simulink model "Galton_Board_v2"  (R2021a)
settings: Solver=ode23t  StartTime=0.0  StopTime=10  MaxStep=1e-3  RelTol=1e-4  AbsTol=1e-4  EnableMultiTasking=on
PreLoadFcn:
  | init_Galton_Board;
values from neighbouring files (symbols this model uses):
  D_ball = 4    [init_Galton_Board.m]
  D_peg = 4    [init_Galton_Board.m]
  H_ground = 200    [init_Galton_Board.m]
  L_peg = 12    [init_Galton_Board.m]
  X = [29.5271269861 43.8447548606 71.2892627183 40.3733262692 -83.4271156395 -32.9172730858 85.8331450424 -78.3400144776 -42.6265382176 30.9682515097 40.2739041017 95.431354449 ... (500 elements, 1x500)]    [results.mat]
undefined symbols (not defined in the file or in its folder): Y, Z
libraries: sm_lib x965, nesl_utility x3
(part 3 of 3)

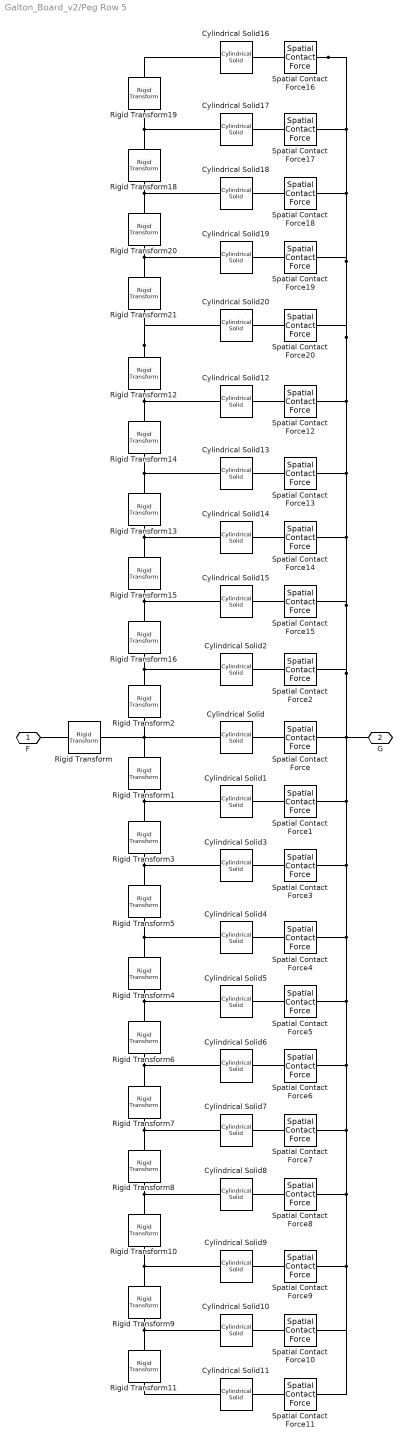
== system Galton_Board_v2/Peg Row 5 ==
  Cylindrical Solid{,1..20} (21 alike) : sm_lib/Body Elements/Cylindrical Solid  GraphicAmbientColor=[0.15 0.15 0.15 1.0]  BasedOnType=Density  CenterOfMass=[0 0 0]  CenterOfMassUnits=m  GraphicDiffuseColor=[0.5 0.5 0.5]  CylinderLength=D*4  CylinderLengthUnits=mm  CylinderRadius=D/2  CylinderRadiusUnits=mm  Density=1000  DensityUnits=kg/m^3  DoExposeReferenceFrame=on  GraphicEmissiveColor=[0.0 0.0 0.0 1.0]  ExportEntireGeometry=on  SerializedFrames=<Frames/>  MarkerShape=Sphere  MarkerSize=10  GraphicType=FromGeometry  InertiaType=CalculateFromGeometry  Mass=1  MassUnits=kg  MomentsOfInertia=[1 1 1]  MomentsOfInertiaUnits=kg*m^2  GraphicOpacity=1.0  ProductsOfInertia=[0 0 0]  ProductsOfInertiaUnits=kg*m^2  GraphicShininess=75  GraphicSpecularColor=[0.5 0.5 0.5 1.0]  GraphicVisPropType=SimpleVisualProperties
  Rigid Transform : sm_lib/Frames and Transforms/Rigid Transform  TranslationMethod=None  TranslationStandardOffset=0  TranslationLengthUnit=m  TranslationStandardAxis=+Z  TranslationCartesianOffset=[0 0 0]  TranslationROffset=0  TranslationROffsetUnits=m  TranslationZOffset=0  TranslationZOffsetUnits=m  TranslationThetaOffset=0  TranslationThetaOffsetUnits=deg  RotationMethod=StandardAxis  RotationAngleUnits=deg  RotationStandardAxis=+X  RotationAngle=90  RotationArbitraryAxis=[0 0 1]  FollAlignAxisA=+X  BaseAlignAxisA=+Y  FollAlignAxisB=+Y  BaseAlignAxisB=+Z  RotationSequenceAxes=FollowerAxes  RotationSequence=XYX  RotationSequenceAngles=[0 0 0]  RotationSequenceAnglesUnits=deg  RotationMatrix=[1 0 0; 0 1 0; 0 0 1]
  Rigid Transform{1..16,18..21} (20 alike) : sm_lib/Frames and Transforms/Rigid Transform  TranslationMethod=StandardAxis  TranslationStandardOffset=L  TranslationLengthUnit=mm  TranslationStandardAxis=+X  TranslationCartesianOffset=[0 0 0]  TranslationROffset=0  TranslationROffsetUnits=m  TranslationZOffset=0  TranslationZOffsetUnits=m  TranslationThetaOffset=0  TranslationThetaOffsetUnits=deg  RotationMethod=None  RotationAngleUnits=deg  RotationStandardAxis=+X  RotationAngle=90  RotationArbitraryAxis=[0 0 1]  FollAlignAxisA=+X  BaseAlignAxisA=+Y  FollAlignAxisB=+Y  BaseAlignAxisB=+Z  RotationSequenceAxes=FollowerAxes  RotationSequence=XYX  RotationSequenceAngles=[0 0 0]  RotationSequenceAnglesUnits=deg  RotationMatrix=[1 0 0; 0 1 0; 0 0 1]
  Spatial Contact Force{,1..20} (21 alike) : sm_lib/Forces and Torques/Spatial Contact Force  CoefficientOfDynamicFriction=0.3  CoefficientOfStaticFriction=0.5  SenseContactBaseRotation=off  SenseContactBaseTranslation=off  NormalDamping=b_scf  NormalDampingUnits=N/(m/s)  SenseContactFollowerRotation=off  SenseContactFollowerTranslation=off  SenseContactSignal=off  NormalStiffness=k_scf  NormalStiffnessUnits=N/m  FrictionalCriticalVelocity=1e-3  FrictionalCriticalVelocityUnits=m/s  ZeroCrossDetectContactStartAndEnd=off  FrictionType=SmoothStickSlip  SenseFrictionalForceMagnitude=off  SenseNormalForceMagnitude=off  NormalForceType=SmoothSpringDamper  SenseNormalVelocity=off  SenseSeparationDistance=off  SenseTangentialVelocity=off  SenseTangentialVelocityMagnitude=off  NormalTransitionRegionWidth=d_scf  NormalTransitionRegionWidthUnits=mm
  F : PMIOPort  Side=Left
  G : PMIOPort  Port=2  Side=Right
  connections:
  Spatial Contact Force19/LConn1 -- Cylindrical Solid19/LConn1
  Spatial Contact Force18/LConn1 -- Cylindrical Solid18/LConn1
  Spatial Contact Force20/LConn1 -- Cylindrical Solid20/LConn1
  Cylindrical Solid17/LConn1 -- Spatial Contact Force17/LConn1
  Spatial Contact Force16/LConn1 -- Cylindrical Solid16/LConn1
  Rigid Transform12/LConn1 -- Cylindrical Solid20/RConn1 -- Rigid Transform21/RConn1
  Rigid Transform20/RConn1 -- Rigid Transform21/LConn1 -- Cylindrical Solid19/RConn1
  Rigid Transform19/RConn1 -- Rigid Transform18/LConn1 -- Cylindrical Solid17/RConn1
  Rigid Transform19/LConn1 -- Cylindrical Solid16/RConn1
  Rigid Transform20/LConn1 -- Rigid Transform18/RConn1 -- Cylindrical Solid18/RConn1
  Spatial Contact Force12/LConn1 -- Cylindrical Solid12/LConn1
  Cylindrical Solid13/LConn1 -- Spatial Contact Force13/LConn1
  Spatial Contact Force14/LConn1 -- Cylindrical Solid14/LConn1
  Spatial Contact Force15/LConn1 -- Cylindrical Solid15/LConn1
  Rigid Transform15/RConn1 -- Rigid Transform16/LConn1 -- Cylindrical Solid15/RConn1
  Rigid Transform15/LConn1 -- Rigid Transform13/RConn1 -- Cylindrical Solid14/RConn1
  Rigid Transform14/RConn1 -- Rigid Transform13/LConn1 -- Cylindrical Solid13/RConn1
  Rigid Transform12/RConn1 -- Rigid Transform14/LConn1 -- Cylindrical Solid12/RConn1
  Spatial Contact Force8/LConn1 -- Cylindrical Solid8/LConn1
  Spatial Contact Force7/LConn1 -- Cylindrical Solid7/LConn1
  Spatial Contact Force10/LConn1 -- Cylindrical Solid10/LConn1
  Rigid Transform11/RConn1 -- Cylindrical Solid11/RConn1
  Cylindrical Solid9/LConn1 -- Spatial Contact Force9/LConn1
  Spatial Contact Force11/LConn1 -- Cylindrical Solid11/LConn1
  Rigid Transform11/LConn1 -- Rigid Transform9/RConn1 -- Cylindrical Solid10/RConn1
  Rigid Transform10/RConn1 -- Rigid Transform9/LConn1 -- Cylindrical Solid9/RConn1
  Rigid Transform8/RConn1 -- Rigid Transform10/LConn1 -- Cylindrical Solid8/RConn1
  Rigid Transform7/RConn1 -- Rigid Transform8/LConn1 -- Cylindrical Solid7/RConn1
  Spatial Contact Force6/LConn1 -- Cylindrical Solid6/LConn1
  Cylindrical Solid4/LConn1 -- Spatial Contact Force4/LConn1
  Rigid Transform7/LConn1 -- Rigid Transform6/RConn1 -- Cylindrical Solid6/RConn1
  Spatial Contact Force5/LConn1 -- Cylindrical Solid5/LConn1
  Rigid Transform4/RConn1 -- Rigid Transform6/LConn1 -- Cylindrical Solid5/RConn1
  Rigid Transform4/LConn1 -- Rigid Transform5/RConn1 -- Cylindrical Solid4/RConn1
  Rigid Transform5/LConn1 -- Rigid Transform3/RConn1 -- Cylindrical Solid3/RConn1
  Spatial Contact Force3/LConn1 -- Cylindrical Solid3/LConn1
  Rigid Transform16/RConn1 -- Cylindrical Solid2/RConn1 -- Rigid Transform2/LConn1
  Spatial Contact Force2/LConn1 -- Cylindrical Solid2/LConn1
  Spatial Contact Force1/LConn1 -- Cylindrical Solid1/LConn1
  Spatial Contact Force16/RConn1 -- Spatial Contact Force17/RConn1 -- Spatial Contact Force18/RConn1 -- Spatial Contact Force19/RConn1 -- Spatial Contact Force20/RConn1 -- Spatial Contact Force15/RConn1 -- Spatial Contact Force2/RConn1 -- Spatial Contact Force/RConn1 -- G/RConn1 -- Spatial Contact Force1/RConn1 -- Spatial Contact Force3/RConn1 -- Spatial Contact Force5/RConn1 -- Spatial Contact Force10/RConn1 -- Spatial Contact Force11/RConn1 -- Spatial Contact Force9/RConn1 -- Spatial Contact Force8/RConn1 -- Spatial Contact Force7/RConn1 -- Spatial Contact Force6/RConn1 -- Spatial Contact Force4/RConn1 -- Spatial Contact Force14/RConn1 -- Spatial Contact Force13/RConn1 -- Spatial Contact Force12/RConn1
  Rigid Transform3/LConn1 -- Rigid Transform1/RConn1 -- Cylindrical Solid1/RConn1
  Cylindrical Solid/LConn1 -- Spatial Contact Force/LConn1
  Rigid Transform/LConn1 -- F/RConn1
  Rigid Transform2/RConn1 -- Rigid Transform1/LConn1 -- Cylindrical Solid/RConn1 -- Rigid Transform/RConn1

== system Galton_Board_v2/Peg Row 6 ==
  Cylindrical Solid{,1..20} (21 alike) : sm_lib/Body Elements/Cylindrical Solid  GraphicAmbientColor=[0.15 0.15 0.15 1.0]  BasedOnType=Density  CenterOfMass=[0 0 0]  CenterOfMassUnits=m  GraphicDiffuseColor=[0.5 0.5 0.5]  CylinderLength=D*4  CylinderLengthUnits=mm  CylinderRadius=D/2  CylinderRadiusUnits=mm  Density=1000  DensityUnits=kg/m^3  DoExposeReferenceFrame=on  GraphicEmissiveColor=[0.0 0.0 0.0 1.0]  ExportEntireGeometry=on  SerializedFrames=<Frames/>  MarkerShape=Sphere  MarkerSize=10  GraphicType=FromGeometry  InertiaType=CalculateFromGeometry  Mass=1  MassUnits=kg  MomentsOfInertia=[1 1 1]  MomentsOfInertiaUnits=kg*m^2  GraphicOpacity=1.0  ProductsOfInertia=[0 0 0]  ProductsOfInertiaUnits=kg*m^2  GraphicShininess=75  GraphicSpecularColor=[0.5 0.5 0.5 1.0]  GraphicVisPropType=SimpleVisualProperties
  Rigid Transform : sm_lib/Frames and Transforms/Rigid Transform  TranslationMethod=None  TranslationStandardOffset=0  TranslationLengthUnit=m  TranslationStandardAxis=+Z  TranslationCartesianOffset=[0 0 0]  TranslationROffset=0  TranslationROffsetUnits=m  TranslationZOffset=0  TranslationZOffsetUnits=m  TranslationThetaOffset=0  TranslationThetaOffsetUnits=deg  RotationMethod=StandardAxis  RotationAngleUnits=deg  RotationStandardAxis=+X  RotationAngle=90  RotationArbitraryAxis=[0 0 1]  FollAlignAxisA=+X  BaseAlignAxisA=+Y  FollAlignAxisB=+Y  BaseAlignAxisB=+Z  RotationSequenceAxes=FollowerAxes  RotationSequence=XYX  RotationSequenceAngles=[0 0 0]  RotationSequenceAnglesUnits=deg  RotationMatrix=[1 0 0; 0 1 0; 0 0 1]
  Rigid Transform{1..16,18..21} (20 alike) : sm_lib/Frames and Transforms/Rigid Transform  TranslationMethod=StandardAxis  TranslationStandardOffset=L  TranslationLengthUnit=mm  TranslationStandardAxis=+X  TranslationCartesianOffset=[0 0 0]  TranslationROffset=0  TranslationROffsetUnits=m  TranslationZOffset=0  TranslationZOffsetUnits=m  TranslationThetaOffset=0  TranslationThetaOffsetUnits=deg  RotationMethod=None  RotationAngleUnits=deg  RotationStandardAxis=+X  RotationAngle=90  RotationArbitraryAxis=[0 0 1]  FollAlignAxisA=+X  BaseAlignAxisA=+Y  FollAlignAxisB=+Y  BaseAlignAxisB=+Z  RotationSequenceAxes=FollowerAxes  RotationSequence=XYX  RotationSequenceAngles=[0 0 0]  RotationSequenceAnglesUnits=deg  RotationMatrix=[1 0 0; 0 1 0; 0 0 1]
  Spatial Contact Force{,1..20} (21 alike) : sm_lib/Forces and Torques/Spatial Contact Force  CoefficientOfDynamicFriction=0.3  CoefficientOfStaticFriction=0.5  SenseContactBaseRotation=off  SenseContactBaseTranslation=off  NormalDamping=b_scf  NormalDampingUnits=N/(m/s)  SenseContactFollowerRotation=off  SenseContactFollowerTranslation=off  SenseContactSignal=off  NormalStiffness=k_scf  NormalStiffnessUnits=N/m  FrictionalCriticalVelocity=1e-3  FrictionalCriticalVelocityUnits=m/s  ZeroCrossDetectContactStartAndEnd=off  FrictionType=SmoothStickSlip  SenseFrictionalForceMagnitude=off  SenseNormalForceMagnitude=off  NormalForceType=SmoothSpringDamper  SenseNormalVelocity=off  SenseSeparationDistance=off  SenseTangentialVelocity=off  SenseTangentialVelocityMagnitude=off  NormalTransitionRegionWidth=d_scf  NormalTransitionRegionWidthUnits=mm
  F : PMIOPort  Side=Left
  G : PMIOPort  Port=2  Side=Right
  connections:
  Spatial Contact Force19/LConn1 -- Cylindrical Solid19/LConn1
  Spatial Contact Force18/LConn1 -- Cylindrical Solid18/LConn1
  Spatial Contact Force20/LConn1 -- Cylindrical Solid20/LConn1
  Cylindrical Solid17/LConn1 -- Spatial Contact Force17/LConn1
  Spatial Contact Force16/LConn1 -- Cylindrical Solid16/LConn1
  Rigid Transform12/LConn1 -- Cylindrical Solid20/RConn1 -- Rigid Transform21/RConn1
  Rigid Transform20/RConn1 -- Rigid Transform21/LConn1 -- Cylindrical Solid19/RConn1
  Rigid Transform19/RConn1 -- Rigid Transform18/LConn1 -- Cylindrical Solid17/RConn1
  Rigid Transform19/LConn1 -- Cylindrical Solid16/RConn1
  Rigid Transform20/LConn1 -- Rigid Transform18/RConn1 -- Cylindrical Solid18/RConn1
  Spatial Contact Force12/LConn1 -- Cylindrical Solid12/LConn1
  Cylindrical Solid13/LConn1 -- Spatial Contact Force13/LConn1
  Spatial Contact Force14/LConn1 -- Cylindrical Solid14/LConn1
  Spatial Contact Force15/LConn1 -- Cylindrical Solid15/LConn1
  Rigid Transform15/RConn1 -- Rigid Transform16/LConn1 -- Cylindrical Solid15/RConn1
  Rigid Transform15/LConn1 -- Rigid Transform13/RConn1 -- Cylindrical Solid14/RConn1
  Rigid Transform14/RConn1 -- Rigid Transform13/LConn1 -- Cylindrical Solid13/RConn1
  Rigid Transform12/RConn1 -- Rigid Transform14/LConn1 -- Cylindrical Solid12/RConn1
  Spatial Contact Force8/LConn1 -- Cylindrical Solid8/LConn1
  Spatial Contact Force7/LConn1 -- Cylindrical Solid7/LConn1
  Spatial Contact Force10/LConn1 -- Cylindrical Solid10/LConn1
  Rigid Transform11/RConn1 -- Cylindrical Solid11/RConn1
  Cylindrical Solid9/LConn1 -- Spatial Contact Force9/LConn1
  Spatial Contact Force11/LConn1 -- Cylindrical Solid11/LConn1
  Rigid Transform11/LConn1 -- Rigid Transform9/RConn1 -- Cylindrical Solid10/RConn1
  Rigid Transform10/RConn1 -- Rigid Transform9/LConn1 -- Cylindrical Solid9/RConn1
  Rigid Transform8/RConn1 -- Rigid Transform10/LConn1 -- Cylindrical Solid8/RConn1
  Rigid Transform7/RConn1 -- Rigid Transform8/LConn1 -- Cylindrical Solid7/RConn1
  Spatial Contact Force6/LConn1 -- Cylindrical Solid6/LConn1
  Cylindrical Solid4/LConn1 -- Spatial Contact Force4/LConn1
  Rigid Transform7/LConn1 -- Rigid Transform6/RConn1 -- Cylindrical Solid6/RConn1
  Spatial Contact Force5/LConn1 -- Cylindrical Solid5/LConn1
  Rigid Transform4/RConn1 -- Rigid Transform6/LConn1 -- Cylindrical Solid5/RConn1
  Rigid Transform4/LConn1 -- Rigid Transform5/RConn1 -- Cylindrical Solid4/RConn1
  Rigid Transform5/LConn1 -- Rigid Transform3/RConn1 -- Cylindrical Solid3/RConn1
  Spatial Contact Force3/LConn1 -- Cylindrical Solid3/LConn1
  Rigid Transform16/RConn1 -- Cylindrical Solid2/RConn1 -- Rigid Transform2/LConn1
  Spatial Contact Force2/LConn1 -- Cylindrical Solid2/LConn1
  Spatial Contact Force1/LConn1 -- Cylindrical Solid1/LConn1
  Spatial Contact Force16/RConn1 -- Spatial Contact Force17/RConn1 -- Spatial Contact Force18/RConn1 -- Spatial Contact Force19/RConn1 -- Spatial Contact Force20/RConn1 -- Spatial Contact Force15/RConn1 -- Spatial Contact Force2/RConn1 -- Spatial Contact Force/RConn1 -- G/RConn1 -- Spatial Contact Force1/RConn1 -- Spatial Contact Force3/RConn1 -- Spatial Contact Force5/RConn1 -- Spatial Contact Force10/RConn1 -- Spatial Contact Force11/RConn1 -- Spatial Contact Force9/RConn1 -- Spatial Contact Force8/RConn1 -- Spatial Contact Force7/RConn1 -- Spatial Contact Force6/RConn1 -- Spatial Contact Force4/RConn1 -- Spatial Contact Force14/RConn1 -- Spatial Contact Force13/RConn1 -- Spatial Contact Force12/RConn1
  Rigid Transform3/LConn1 -- Rigid Transform1/RConn1 -- Cylindrical Solid1/RConn1
  Cylindrical Solid/LConn1 -- Spatial Contact Force/LConn1
  Rigid Transform/LConn1 -- F/RConn1
  Rigid Transform2/RConn1 -- Rigid Transform1/LConn1 -- Cylindrical Solid/RConn1 -- Rigid Transform/RConn1

== system Galton_Board_v2/Peg Row 7 ==
  Cylindrical Solid{,1..20} (21 alike) : sm_lib/Body Elements/Cylindrical Solid  GraphicAmbientColor=[0.15 0.15 0.15 1.0]  BasedOnType=Density  CenterOfMass=[0 0 0]  CenterOfMassUnits=m  GraphicDiffuseColor=[0.5 0.5 0.5]  CylinderLength=D*4  CylinderLengthUnits=mm  CylinderRadius=D/2  CylinderRadiusUnits=mm  Density=1000  DensityUnits=kg/m^3  DoExposeReferenceFrame=on  GraphicEmissiveColor=[0.0 0.0 0.0 1.0]  ExportEntireGeometry=on  SerializedFrames=<Frames/>  MarkerShape=Sphere  MarkerSize=10  GraphicType=FromGeometry  InertiaType=CalculateFromGeometry  Mass=1  MassUnits=kg  MomentsOfInertia=[1 1 1]  MomentsOfInertiaUnits=kg*m^2  GraphicOpacity=1.0  ProductsOfInertia=[0 0 0]  ProductsOfInertiaUnits=kg*m^2  GraphicShininess=75  GraphicSpecularColor=[0.5 0.5 0.5 1.0]  GraphicVisPropType=SimpleVisualProperties
  Rigid Transform : sm_lib/Frames and Transforms/Rigid Transform  TranslationMethod=None  TranslationStandardOffset=0  TranslationLengthUnit=m  TranslationStandardAxis=+Z  TranslationCartesianOffset=[0 0 0]  TranslationROffset=0  TranslationROffsetUnits=m  TranslationZOffset=0  TranslationZOffsetUnits=m  TranslationThetaOffset=0  TranslationThetaOffsetUnits=deg  RotationMethod=StandardAxis  RotationAngleUnits=deg  RotationStandardAxis=+X  RotationAngle=90  RotationArbitraryAxis=[0 0 1]  FollAlignAxisA=+X  BaseAlignAxisA=+Y  FollAlignAxisB=+Y  BaseAlignAxisB=+Z  RotationSequenceAxes=FollowerAxes  RotationSequence=XYX  RotationSequenceAngles=[0 0 0]  RotationSequenceAnglesUnits=deg  RotationMatrix=[1 0 0; 0 1 0; 0 0 1]
  Rigid Transform{1..16,18..21} (20 alike) : sm_lib/Frames and Transforms/Rigid Transform  TranslationMethod=StandardAxis  TranslationStandardOffset=L  TranslationLengthUnit=mm  TranslationStandardAxis=+X  TranslationCartesianOffset=[0 0 0]  TranslationROffset=0  TranslationROffsetUnits=m  TranslationZOffset=0  TranslationZOffsetUnits=m  TranslationThetaOffset=0  TranslationThetaOffsetUnits=deg  RotationMethod=None  RotationAngleUnits=deg  RotationStandardAxis=+X  RotationAngle=90  RotationArbitraryAxis=[0 0 1]  FollAlignAxisA=+X  BaseAlignAxisA=+Y  FollAlignAxisB=+Y  BaseAlignAxisB=+Z  RotationSequenceAxes=FollowerAxes  RotationSequence=XYX  RotationSequenceAngles=[0 0 0]  RotationSequenceAnglesUnits=deg  RotationMatrix=[1 0 0; 0 1 0; 0 0 1]
  Spatial Contact Force{,1..20} (21 alike) : sm_lib/Forces and Torques/Spatial Contact Force  CoefficientOfDynamicFriction=0.3  CoefficientOfStaticFriction=0.5  SenseContactBaseRotation=off  SenseContactBaseTranslation=off  NormalDamping=b_scf  NormalDampingUnits=N/(m/s)  SenseContactFollowerRotation=off  SenseContactFollowerTranslation=off  SenseContactSignal=off  NormalStiffness=k_scf  NormalStiffnessUnits=N/m  FrictionalCriticalVelocity=1e-3  FrictionalCriticalVelocityUnits=m/s  ZeroCrossDetectContactStartAndEnd=off  FrictionType=SmoothStickSlip  SenseFrictionalForceMagnitude=off  SenseNormalForceMagnitude=off  NormalForceType=SmoothSpringDamper  SenseNormalVelocity=off  SenseSeparationDistance=off  SenseTangentialVelocity=off  SenseTangentialVelocityMagnitude=off  NormalTransitionRegionWidth=d_scf  NormalTransitionRegionWidthUnits=mm
  F : PMIOPort  Side=Left
  G : PMIOPort  Port=2  Side=Right
  connections:
  Rigid Transform/RConn1 -- Cylindrical Solid/RConn1 -- Rigid Transform1/LConn1 -- Rigid Transform2/RConn1
  Rigid Transform/LConn1 -- F/RConn1
  Cylindrical Solid/LConn1 -- Spatial Contact Force/LConn1
  Cylindrical Solid1/RConn1 -- Rigid Transform1/RConn1 -- Rigid Transform3/LConn1
  Spatial Contact Force12/RConn1 -- Spatial Contact Force13/RConn1 -- Spatial Contact Force14/RConn1 -- Spatial Contact Force4/RConn1 -- Spatial Contact Force6/RConn1 -- Spatial Contact Force7/RConn1 -- Spatial Contact Force8/RConn1 -- Spatial Contact Force9/RConn1 -- Spatial Contact Force11/RConn1 -- Spatial Contact Force10/RConn1 -- Spatial Contact Force5/RConn1 -- Spatial Contact Force3/RConn1 -- Spatial Contact Force1/RConn1 -- G/RConn1 -- Spatial Contact Force/RConn1 -- Spatial Contact Force2/RConn1 -- Spatial Contact Force15/RConn1 -- Spatial Contact Force20/RConn1 -- Spatial Contact Force19/RConn1 -- Spatial Contact Force18/RConn1 -- Spatial Contact Force17/RConn1 -- Spatial Contact Force16/RConn1
  Spatial Contact Force1/LConn1 -- Cylindrical Solid1/LConn1
  Spatial Contact Force2/LConn1 -- Cylindrical Solid2/LConn1
  Rigid Transform2/LConn1 -- Cylindrical Solid2/RConn1 -- Rigid Transform16/RConn1
  Spatial Contact Force3/LConn1 -- Cylindrical Solid3/LConn1
  Cylindrical Solid3/RConn1 -- Rigid Transform3/RConn1 -- Rigid Transform5/LConn1
  Cylindrical Solid4/RConn1 -- Rigid Transform5/RConn1 -- Rigid Transform4/LConn1
  Cylindrical Solid5/RConn1 -- Rigid Transform6/LConn1 -- Rigid Transform4/RConn1
  Spatial Contact Force5/LConn1 -- Cylindrical Solid5/LConn1
  Cylindrical Solid6/RConn1 -- Rigid Transform6/RConn1 -- Rigid Transform7/LConn1
  Cylindrical Solid4/LConn1 -- Spatial Contact Force4/LConn1
  Spatial Contact Force6/LConn1 -- Cylindrical Solid6/LConn1
  Cylindrical Solid7/RConn1 -- Rigid Transform8/LConn1 -- Rigid Transform7/RConn1
  Cylindrical Solid8/RConn1 -- Rigid Transform10/LConn1 -- Rigid Transform8/RConn1
  Cylindrical Solid9/RConn1 -- Rigid Transform9/LConn1 -- Rigid Transform10/RConn1
  Cylindrical Solid10/RConn1 -- Rigid Transform9/RConn1 -- Rigid Transform11/LConn1
  Spatial Contact Force11/LConn1 -- Cylindrical Solid11/LConn1
  Cylindrical Solid9/LConn1 -- Spatial Contact Force9/LConn1
  Rigid Transform11/RConn1 -- Cylindrical Solid11/RConn1
  Spatial Contact Force10/LConn1 -- Cylindrical Solid10/LConn1
  Spatial Contact Force7/LConn1 -- Cylindrical Solid7/LConn1
  Spatial Contact Force8/LConn1 -- Cylindrical Solid8/LConn1
  Cylindrical Solid12/RConn1 -- Rigid Transform14/LConn1 -- Rigid Transform12/RConn1
  Cylindrical Solid13/RConn1 -- Rigid Transform13/LConn1 -- Rigid Transform14/RConn1
  Cylindrical Solid14/RConn1 -- Rigid Transform13/RConn1 -- Rigid Transform15/LConn1
  Cylindrical Solid15/RConn1 -- Rigid Transform16/LConn1 -- Rigid Transform15/RConn1
  Spatial Contact Force15/LConn1 -- Cylindrical Solid15/LConn1
  Spatial Contact Force14/LConn1 -- Cylindrical Solid14/LConn1
  Cylindrical Solid13/LConn1 -- Spatial Contact Force13/LConn1
  Spatial Contact Force12/LConn1 -- Cylindrical Solid12/LConn1
  Cylindrical Solid18/RConn1 -- Rigid Transform18/RConn1 -- Rigid Transform20/LConn1
  Rigid Transform19/LConn1 -- Cylindrical Solid16/RConn1
  Cylindrical Solid17/RConn1 -- Rigid Transform18/LConn1 -- Rigid Transform19/RConn1
  Cylindrical Solid19/RConn1 -- Rigid Transform21/LConn1 -- Rigid Transform20/RConn1
  Rigid Transform21/RConn1 -- Cylindrical Solid20/RConn1 -- Rigid Transform12/LConn1
  Spatial Contact Force16/LConn1 -- Cylindrical Solid16/LConn1
  Cylindrical Solid17/LConn1 -- Spatial Contact Force17/LConn1
  Spatial Contact Force20/LConn1 -- Cylindrical Solid20/LConn1
  Spatial Contact Force18/LConn1 -- Cylindrical Solid18/LConn1
  Spatial Contact Force19/LConn1 -- Cylindrical Solid19/LConn1

== system Galton_Board_v2/Peg Row 8 ==
  Cylindrical Solid{,1..20} (21 alike) : sm_lib/Body Elements/Cylindrical Solid  GraphicAmbientColor=[0.15 0.15 0.15 1.0]  BasedOnType=Density  CenterOfMass=[0 0 0]  CenterOfMassUnits=m  GraphicDiffuseColor=[0.5 0.5 0.5]  CylinderLength=D*4  CylinderLengthUnits=mm  CylinderRadius=D/2  CylinderRadiusUnits=mm  Density=1000  DensityUnits=kg/m^3  DoExposeReferenceFrame=on  GraphicEmissiveColor=[0.0 0.0 0.0 1.0]  ExportEntireGeometry=on  SerializedFrames=<Frames/>  MarkerShape=Sphere  MarkerSize=10  GraphicType=FromGeometry  InertiaType=CalculateFromGeometry  Mass=1  MassUnits=kg  MomentsOfInertia=[1 1 1]  MomentsOfInertiaUnits=kg*m^2  GraphicOpacity=1.0  ProductsOfInertia=[0 0 0]  ProductsOfInertiaUnits=kg*m^2  GraphicShininess=75  GraphicSpecularColor=[0.5 0.5 0.5 1.0]  GraphicVisPropType=SimpleVisualProperties
  Rigid Transform : sm_lib/Frames and Transforms/Rigid Transform  TranslationMethod=None  TranslationStandardOffset=0  TranslationLengthUnit=m  TranslationStandardAxis=+Z  TranslationCartesianOffset=[0 0 0]  TranslationROffset=0  TranslationROffsetUnits=m  TranslationZOffset=0  TranslationZOffsetUnits=m  TranslationThetaOffset=0  TranslationThetaOffsetUnits=deg  RotationMethod=StandardAxis  RotationAngleUnits=deg  RotationStandardAxis=+X  RotationAngle=90  RotationArbitraryAxis=[0 0 1]  FollAlignAxisA=+X  BaseAlignAxisA=+Y  FollAlignAxisB=+Y  BaseAlignAxisB=+Z  RotationSequenceAxes=FollowerAxes  RotationSequence=XYX  RotationSequenceAngles=[0 0 0]  RotationSequenceAnglesUnits=deg  RotationMatrix=[1 0 0; 0 1 0; 0 0 1]
  Rigid Transform{1..16,18..21} (20 alike) : sm_lib/Frames and Transforms/Rigid Transform  TranslationMethod=StandardAxis  TranslationStandardOffset=L  TranslationLengthUnit=mm  TranslationStandardAxis=+X  TranslationCartesianOffset=[0 0 0]  TranslationROffset=0  TranslationROffsetUnits=m  TranslationZOffset=0  TranslationZOffsetUnits=m  TranslationThetaOffset=0  TranslationThetaOffsetUnits=deg  RotationMethod=None  RotationAngleUnits=deg  RotationStandardAxis=+X  RotationAngle=90  RotationArbitraryAxis=[0 0 1]  FollAlignAxisA=+X  BaseAlignAxisA=+Y  FollAlignAxisB=+Y  BaseAlignAxisB=+Z  RotationSequenceAxes=FollowerAxes  RotationSequence=XYX  RotationSequenceAngles=[0 0 0]  RotationSequenceAnglesUnits=deg  RotationMatrix=[1 0 0; 0 1 0; 0 0 1]
  Spatial Contact Force{,1..20} (21 alike) : sm_lib/Forces and Torques/Spatial Contact Force  CoefficientOfDynamicFriction=0.3  CoefficientOfStaticFriction=0.5  SenseContactBaseRotation=off  SenseContactBaseTranslation=off  NormalDamping=b_scf  NormalDampingUnits=N/(m/s)  SenseContactFollowerRotation=off  SenseContactFollowerTranslation=off  SenseContactSignal=off  NormalStiffness=k_scf  NormalStiffnessUnits=N/m  FrictionalCriticalVelocity=1e-3  FrictionalCriticalVelocityUnits=m/s  ZeroCrossDetectContactStartAndEnd=off  FrictionType=SmoothStickSlip  SenseFrictionalForceMagnitude=off  SenseNormalForceMagnitude=off  NormalForceType=SmoothSpringDamper  SenseNormalVelocity=off  SenseSeparationDistance=off  SenseTangentialVelocity=off  SenseTangentialVelocityMagnitude=off  NormalTransitionRegionWidth=d_scf  NormalTransitionRegionWidthUnits=mm
  F : PMIOPort  Side=Left
  G : PMIOPort  Port=2  Side=Right
  connections:
  Rigid Transform/RConn1 -- Cylindrical Solid/RConn1 -- Rigid Transform1/LConn1 -- Rigid Transform2/RConn1
  Rigid Transform/LConn1 -- F/RConn1
  Cylindrical Solid/LConn1 -- Spatial Contact Force/LConn1
  Cylindrical Solid1/RConn1 -- Rigid Transform1/RConn1 -- Rigid Transform3/LConn1
  Spatial Contact Force12/RConn1 -- Spatial Contact Force13/RConn1 -- Spatial Contact Force14/RConn1 -- Spatial Contact Force4/RConn1 -- Spatial Contact Force6/RConn1 -- Spatial Contact Force7/RConn1 -- Spatial Contact Force8/RConn1 -- Spatial Contact Force9/RConn1 -- Spatial Contact Force11/RConn1 -- Spatial Contact Force10/RConn1 -- Spatial Contact Force5/RConn1 -- Spatial Contact Force3/RConn1 -- Spatial Contact Force1/RConn1 -- G/RConn1 -- Spatial Contact Force/RConn1 -- Spatial Contact Force2/RConn1 -- Spatial Contact Force15/RConn1 -- Spatial Contact Force20/RConn1 -- Spatial Contact Force19/RConn1 -- Spatial Contact Force18/RConn1 -- Spatial Contact Force17/RConn1 -- Spatial Contact Force16/RConn1
  Spatial Contact Force1/LConn1 -- Cylindrical Solid1/LConn1
  Spatial Contact Force2/LConn1 -- Cylindrical Solid2/LConn1
  Rigid Transform2/LConn1 -- Cylindrical Solid2/RConn1 -- Rigid Transform16/RConn1
  Spatial Contact Force3/LConn1 -- Cylindrical Solid3/LConn1
  Cylindrical Solid3/RConn1 -- Rigid Transform3/RConn1 -- Rigid Transform5/LConn1
  Cylindrical Solid4/RConn1 -- Rigid Transform5/RConn1 -- Rigid Transform4/LConn1
  Cylindrical Solid5/RConn1 -- Rigid Transform6/LConn1 -- Rigid Transform4/RConn1
  Spatial Contact Force5/LConn1 -- Cylindrical Solid5/LConn1
  Cylindrical Solid6/RConn1 -- Rigid Transform6/RConn1 -- Rigid Transform7/LConn1
  Cylindrical Solid4/LConn1 -- Spatial Contact Force4/LConn1
  Spatial Contact Force6/LConn1 -- Cylindrical Solid6/LConn1
  Cylindrical Solid7/RConn1 -- Rigid Transform8/LConn1 -- Rigid Transform7/RConn1
  Cylindrical Solid8/RConn1 -- Rigid Transform10/LConn1 -- Rigid Transform8/RConn1
  Cylindrical Solid9/RConn1 -- Rigid Transform9/LConn1 -- Rigid Transform10/RConn1
  Cylindrical Solid10/RConn1 -- Rigid Transform9/RConn1 -- Rigid Transform11/LConn1
  Spatial Contact Force11/LConn1 -- Cylindrical Solid11/LConn1
  Cylindrical Solid9/LConn1 -- Spatial Contact Force9/LConn1
  Rigid Transform11/RConn1 -- Cylindrical Solid11/RConn1
  Spatial Contact Force10/LConn1 -- Cylindrical Solid10/LConn1
  Spatial Contact Force7/LConn1 -- Cylindrical Solid7/LConn1
  Spatial Contact Force8/LConn1 -- Cylindrical Solid8/LConn1
  Cylindrical Solid12/RConn1 -- Rigid Transform14/LConn1 -- Rigid Transform12/RConn1
  Cylindrical Solid13/RConn1 -- Rigid Transform13/LConn1 -- Rigid Transform14/RConn1
  Cylindrical Solid14/RConn1 -- Rigid Transform13/RConn1 -- Rigid Transform15/LConn1
  Cylindrical Solid15/RConn1 -- Rigid Transform16/LConn1 -- Rigid Transform15/RConn1
  Spatial Contact Force15/LConn1 -- Cylindrical Solid15/LConn1
  Spatial Contact Force14/LConn1 -- Cylindrical Solid14/LConn1
  Cylindrical Solid13/LConn1 -- Spatial Contact Force13/LConn1
  Spatial Contact Force12/LConn1 -- Cylindrical Solid12/LConn1
  Cylindrical Solid18/RConn1 -- Rigid Transform18/RConn1 -- Rigid Transform20/LConn1
  Rigid Transform19/LConn1 -- Cylindrical Solid16/RConn1
  Cylindrical Solid17/RConn1 -- Rigid Transform18/LConn1 -- Rigid Transform19/RConn1
  Cylindrical Solid19/RConn1 -- Rigid Transform21/LConn1 -- Rigid Transform20/RConn1
  Rigid Transform21/RConn1 -- Cylindrical Solid20/RConn1 -- Rigid Transform12/LConn1
  Spatial Contact Force16/LConn1 -- Cylindrical Solid16/LConn1
  Cylindrical Solid17/LConn1 -- Spatial Contact Force17/LConn1
  Spatial Contact Force20/LConn1 -- Cylindrical Solid20/LConn1
  Spatial Contact Force18/LConn1 -- Cylindrical Solid18/LConn1
  Spatial Contact Force19/LConn1 -- Cylindrical Solid19/LConn1

== system Galton_Board_v2/Peg Row 9 ==
  Cylindrical Solid{,1..20} (21 alike) : sm_lib/Body Elements/Cylindrical Solid  GraphicAmbientColor=[0.15 0.15 0.15 1.0]  BasedOnType=Density  CenterOfMass=[0 0 0]  CenterOfMassUnits=m  GraphicDiffuseColor=[0.5 0.5 0.5]  CylinderLength=D*4  CylinderLengthUnits=mm  CylinderRadius=D/2  CylinderRadiusUnits=mm  Density=1000  DensityUnits=kg/m^3  DoExposeReferenceFrame=on  GraphicEmissiveColor=[0.0 0.0 0.0 1.0]  ExportEntireGeometry=on  SerializedFrames=<Frames/>  MarkerShape=Sphere  MarkerSize=10  GraphicType=FromGeometry  InertiaType=CalculateFromGeometry  Mass=1  MassUnits=kg  MomentsOfInertia=[1 1 1]  MomentsOfInertiaUnits=kg*m^2  GraphicOpacity=1.0  ProductsOfInertia=[0 0 0]  ProductsOfInertiaUnits=kg*m^2  GraphicShininess=75  GraphicSpecularColor=[0.5 0.5 0.5 1.0]  GraphicVisPropType=SimpleVisualProperties
  Rigid Transform : sm_lib/Frames and Transforms/Rigid Transform  TranslationMethod=None  TranslationStandardOffset=0  TranslationLengthUnit=m  TranslationStandardAxis=+Z  TranslationCartesianOffset=[0 0 0]  TranslationROffset=0  TranslationROffsetUnits=m  TranslationZOffset=0  TranslationZOffsetUnits=m  TranslationThetaOffset=0  TranslationThetaOffsetUnits=deg  RotationMethod=StandardAxis  RotationAngleUnits=deg  RotationStandardAxis=+X  RotationAngle=90  RotationArbitraryAxis=[0 0 1]  FollAlignAxisA=+X  BaseAlignAxisA=+Y  FollAlignAxisB=+Y  BaseAlignAxisB=+Z  RotationSequenceAxes=FollowerAxes  RotationSequence=XYX  RotationSequenceAngles=[0 0 0]  RotationSequenceAnglesUnits=deg  RotationMatrix=[1 0 0; 0 1 0; 0 0 1]
  Rigid Transform{1..16,18..21} (20 alike) : sm_lib/Frames and Transforms/Rigid Transform  TranslationMethod=StandardAxis  TranslationStandardOffset=L  TranslationLengthUnit=mm  TranslationStandardAxis=+X  TranslationCartesianOffset=[0 0 0]  TranslationROffset=0  TranslationROffsetUnits=m  TranslationZOffset=0  TranslationZOffsetUnits=m  TranslationThetaOffset=0  TranslationThetaOffsetUnits=deg  RotationMethod=None  RotationAngleUnits=deg  RotationStandardAxis=+X  RotationAngle=90  RotationArbitraryAxis=[0 0 1]  FollAlignAxisA=+X  BaseAlignAxisA=+Y  FollAlignAxisB=+Y  BaseAlignAxisB=+Z  RotationSequenceAxes=FollowerAxes  RotationSequence=XYX  RotationSequenceAngles=[0 0 0]  RotationSequenceAnglesUnits=deg  RotationMatrix=[1 0 0; 0 1 0; 0 0 1]
  Spatial Contact Force{,1..20} (21 alike) : sm_lib/Forces and Torques/Spatial Contact Force  CoefficientOfDynamicFriction=0.3  CoefficientOfStaticFriction=0.5  SenseContactBaseRotation=off  SenseContactBaseTranslation=off  NormalDamping=b_scf  NormalDampingUnits=N/(m/s)  SenseContactFollowerRotation=off  SenseContactFollowerTranslation=off  SenseContactSignal=off  NormalStiffness=k_scf  NormalStiffnessUnits=N/m  FrictionalCriticalVelocity=1e-3  FrictionalCriticalVelocityUnits=m/s  ZeroCrossDetectContactStartAndEnd=off  FrictionType=SmoothStickSlip  SenseFrictionalForceMagnitude=off  SenseNormalForceMagnitude=off  NormalForceType=SmoothSpringDamper  SenseNormalVelocity=off  SenseSeparationDistance=off  SenseTangentialVelocity=off  SenseTangentialVelocityMagnitude=off  NormalTransitionRegionWidth=d_scf  NormalTransitionRegionWidthUnits=mm
  F : PMIOPort  Side=Left
  G : PMIOPort  Port=2  Side=Right
  connections:
  Spatial Contact Force19/LConn1 -- Cylindrical Solid19/LConn1
  Spatial Contact Force18/LConn1 -- Cylindrical Solid18/LConn1
  Spatial Contact Force20/LConn1 -- Cylindrical Solid20/LConn1
  Cylindrical Solid17/LConn1 -- Spatial Contact Force17/LConn1
  Spatial Contact Force16/LConn1 -- Cylindrical Solid16/LConn1
  Rigid Transform12/LConn1 -- Cylindrical Solid20/RConn1 -- Rigid Transform21/RConn1
  Rigid Transform20/RConn1 -- Rigid Transform21/LConn1 -- Cylindrical Solid19/RConn1
  Rigid Transform19/RConn1 -- Rigid Transform18/LConn1 -- Cylindrical Solid17/RConn1
  Rigid Transform19/LConn1 -- Cylindrical Solid16/RConn1
  Rigid Transform20/LConn1 -- Rigid Transform18/RConn1 -- Cylindrical Solid18/RConn1
  Spatial Contact Force12/LConn1 -- Cylindrical Solid12/LConn1
  Cylindrical Solid13/LConn1 -- Spatial Contact Force13/LConn1
  Spatial Contact Force14/LConn1 -- Cylindrical Solid14/LConn1
  Spatial Contact Force15/LConn1 -- Cylindrical Solid15/LConn1
  Rigid Transform15/RConn1 -- Rigid Transform16/LConn1 -- Cylindrical Solid15/RConn1
  Rigid Transform15/LConn1 -- Rigid Transform13/RConn1 -- Cylindrical Solid14/RConn1
  Rigid Transform14/RConn1 -- Rigid Transform13/LConn1 -- Cylindrical Solid13/RConn1
  Rigid Transform12/RConn1 -- Rigid Transform14/LConn1 -- Cylindrical Solid12/RConn1
  Spatial Contact Force8/LConn1 -- Cylindrical Solid8/LConn1
  Spatial Contact Force7/LConn1 -- Cylindrical Solid7/LConn1
  Spatial Contact Force10/LConn1 -- Cylindrical Solid10/LConn1
  Rigid Transform11/RConn1 -- Cylindrical Solid11/RConn1
  Cylindrical Solid9/LConn1 -- Spatial Contact Force9/LConn1
  Spatial Contact Force11/LConn1 -- Cylindrical Solid11/LConn1
  Rigid Transform11/LConn1 -- Rigid Transform9/RConn1 -- Cylindrical Solid10/RConn1
  Rigid Transform10/RConn1 -- Rigid Transform9/LConn1 -- Cylindrical Solid9/RConn1
  Rigid Transform8/RConn1 -- Rigid Transform10/LConn1 -- Cylindrical Solid8/RConn1
  Rigid Transform7/RConn1 -- Rigid Transform8/LConn1 -- Cylindrical Solid7/RConn1
  Spatial Contact Force6/LConn1 -- Cylindrical Solid6/LConn1
  Cylindrical Solid4/LConn1 -- Spatial Contact Force4/LConn1
  Rigid Transform7/LConn1 -- Rigid Transform6/RConn1 -- Cylindrical Solid6/RConn1
  Spatial Contact Force5/LConn1 -- Cylindrical Solid5/LConn1
  Rigid Transform4/RConn1 -- Rigid Transform6/LConn1 -- Cylindrical Solid5/RConn1
  Rigid Transform4/LConn1 -- Rigid Transform5/RConn1 -- Cylindrical Solid4/RConn1
  Rigid Transform5/LConn1 -- Rigid Transform3/RConn1 -- Cylindrical Solid3/RConn1
  Spatial Contact Force3/LConn1 -- Cylindrical Solid3/LConn1
  Rigid Transform16/RConn1 -- Cylindrical Solid2/RConn1 -- Rigid Transform2/LConn1
  Spatial Contact Force2/LConn1 -- Cylindrical Solid2/LConn1
  Spatial Contact Force1/LConn1 -- Cylindrical Solid1/LConn1
  Spatial Contact Force16/RConn1 -- Spatial Contact Force17/RConn1 -- Spatial Contact Force18/RConn1 -- Spatial Contact Force19/RConn1 -- Spatial Contact Force20/RConn1 -- Spatial Contact Force15/RConn1 -- Spatial Contact Force2/RConn1 -- Spatial Contact Force/RConn1 -- G/RConn1 -- Spatial Contact Force1/RConn1 -- Spatial Contact Force3/RConn1 -- Spatial Contact Force5/RConn1 -- Spatial Contact Force10/RConn1 -- Spatial Contact Force11/RConn1 -- Spatial Contact Force9/RConn1 -- Spatial Contact Force8/RConn1 -- Spatial Contact Force7/RConn1 -- Spatial Contact Force6/RConn1 -- Spatial Contact Force4/RConn1 -- Spatial Contact Force14/RConn1 -- Spatial Contact Force13/RConn1 -- Spatial Contact Force12/RConn1
  Rigid Transform3/LConn1 -- Rigid Transform1/RConn1 -- Cylindrical Solid1/RConn1
  Cylindrical Solid/LConn1 -- Spatial Contact Force/LConn1
  Rigid Transform/LConn1 -- F/RConn1
  Rigid Transform2/RConn1 -- Rigid Transform1/LConn1 -- Cylindrical Solid/RConn1 -- Rigid Transform/RConn1
